simulink model "TRAS_DevDriv"  (R2012b)
settings: Solver=ode4  StartTime=0.0  StopTime=60  FixedStep=0.01  RelTol=1e-3
settings Model: SimulationMode=external  ExtModeTrigDuration=10000  Creator=user  LastModifiedBy=inteco
settings DataIOCC: SignalLoggingSaveFormat=ModelDataLogs
settings DebuggingCC: FcnCallInpInsideContextMsg=UseLocalSettings
settings RTWCC: SystemTargetFile=rtcon_tras_usb2.tlc  TemplateMakefile=rtcon_tras_vc_usb2_x64.tmf  Description=TRAS RTDAC/USB2 (Visual C/C++)  ProcessScript=rtcon_tras_usb2_make_rtw_hook
settings STFCustomTargetCC: CodeReplacementLibrary=ANSI_C  ModelReferenceCompliant=off  GeneratePreprocessorConditionals=Disable all  CombineOutputUpdateFcns=on  MatFileLogging=on  GRTInterface=off  SystemTargetFile=rtcon_tras_usb2.tlc
settings GRTTargetCC: ModelReferenceCompliant=off  ParMdlRefBuildCompliant=off  CompOptLevelCompliant=off  ConcurrentExecutionCompliant=off  ExtMode=on  ExtModeMexFile=rtcon_ext_comm

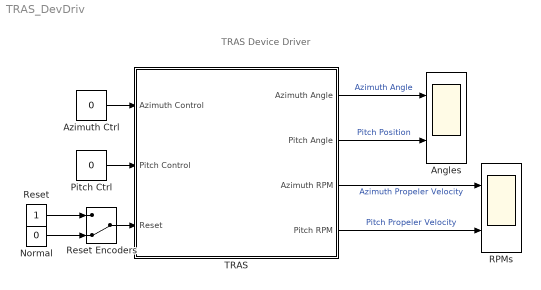
== system TRAS_DevDriv ==
  note: TRAS Device Driver
  Angles : Scope  NumInputPorts=2
      settings: TimeRange=30  YMin=-0.02~-0.1  YMax=0.0025~1  SaveName=SD1  MaxDataPoints=12000
  Azimuth Ctrl : Constant  Value=0
  Normal : Constant  Value=0
  Pitch Ctrl : Constant  Value=0
  RPMs : Scope  NumInputPorts=2
      settings: TimeRange=30  YMin=-20~-400  YMax=0~500  SaveName=SD  MaxDataPoints=12000
  Reset : Constant
  Reset Encoders : ManualSwitch  CurrentSetting=0
  TRAS : Subsystem
      mask Display: image(imread('Tras.JPG'))
  wires:
  TRAS/1(Azimuth Angle) -> Angles/1  "Azimuth Angle"
  TRAS/2(Pitch Angle) -> Angles/2  "Pitch Position"
  Azimuth Ctrl/1 -> TRAS/1(Azimuth Control)
  Pitch Ctrl/1 -> TRAS/2(Pitch Control)
  TRAS/3(Azimuth RPM) -> RPMs/1  "Azimuth Propeler Velocity"
  TRAS/4(Pitch RPM) -> RPMs/2  "Pitch Propeler Velocity"
  Normal/1 -> Reset Encoders/2
  Reset/1 -> Reset Encoders/1
  Reset Encoders/1 -> TRAS/3(Reset)

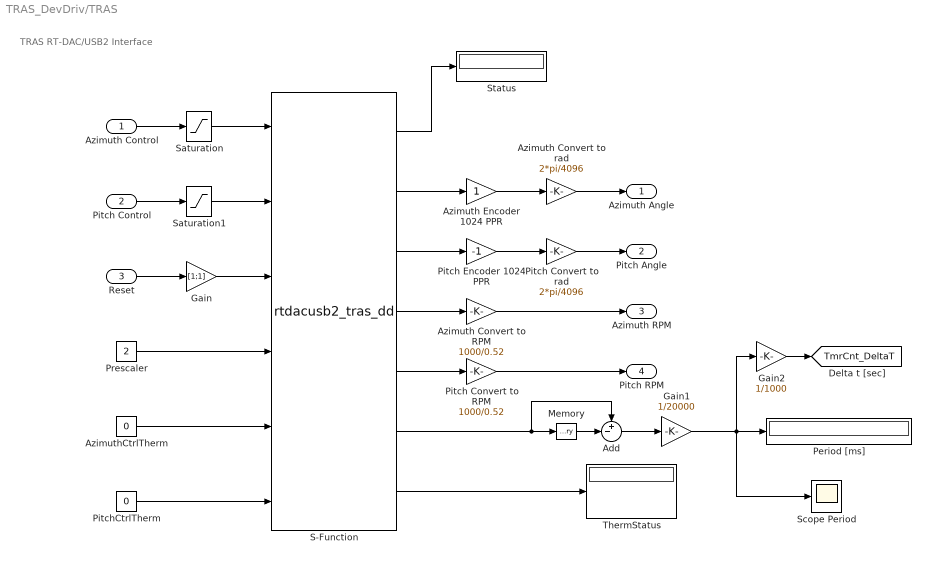
== system TRAS_DevDriv/TRAS ==
  note: TRAS RT-DAC/USB2
      | Interface
  Azimuth Control : Inport
  Pitch Control : Inport  Port=2
  Reset : Inport  Port=3
  Add : Sum  Inputs=+-|
  Azimuth Convert to RPM : Gain  Gain=1000/0.52  SaturateOnIntegerOverflow=on  OutDataTypeStr=Inherit: Same as input  ParamDataTypeStr=Inherit: Same as input
  Azimuth Convert to rad : Gain  Gain=2*pi/4096  SaturateOnIntegerOverflow=on  OutDataTypeStr=Inherit: Same as input  ParamDataTypeStr=Inherit: Same as input
  Azimuth Encoder 1024 PPR : Gain  SaturateOnIntegerOverflow=on  OutDataTypeStr=Inherit: Same as input  ParamDataTypeStr=Inherit: Same as input
  AzimuthCtrlTherm : Constant  Value=0
  Gain : Gain  Gain=[1;1]
  Gain1 : Gain  Gain=1/20000
  Gain2 : Gain  Gain=1/1000
  Memory : Memory
  Period [ms] : Display
  Pitch Convert to RPM : Gain  Gain=1000/0.52  SaturateOnIntegerOverflow=on  OutDataTypeStr=Inherit: Same as input  ParamDataTypeStr=Inherit: Same as input
  Pitch Convert to rad : Gain  Gain=2*pi/4096  SaturateOnIntegerOverflow=on  OutDataTypeStr=Inherit: Same as input  ParamDataTypeStr=Inherit: Same as input
  Pitch Encoder 1024 PPR : Gain  Gain=-1  SaturateOnIntegerOverflow=on  OutDataTypeStr=Inherit: Same as input  ParamDataTypeStr=Inherit: Same as input
  PitchCtrlTherm : Constant  Value=0
  Prescaler : Constant  Value=2
  S-Function : S-Function  FunctionName=rtdacusb2_tras_dd  Parameters=1, 0.01  EnableBusSupport=off
  Saturation : Saturate  UpperLimit=1  LowerLimit=-1
  Saturation1 : Saturate  UpperLimit=1  LowerLimit=-1
  Scope Period : Scope
      settings: TimeRange=30  YMin=0  YMax=6.5e+008
  Status : Display
  ThermStatus : Display
  Azimuth Angle : Outport
  Pitch Angle : Outport  Port=2
  Azimuth RPM : Outport  Port=3
  Pitch RPM : Outport  Port=4
  tag scope: TmrCnt_DeltaT=global
  wires:
  Azimuth Control/1 -> Saturation/1
  Pitch Control/1 -> Saturation1/1
  Reset/1 -> Gain/1
  Prescaler/1 -> S-Function/4
  AzimuthCtrlTherm/1 -> S-Function/5
  PitchCtrlTherm/1 -> S-Function/6
  Saturation/1 -> S-Function/1
  Saturation1/1 -> S-Function/2
  Gain/1 -> S-Function/3
  S-Function/1 -> Status/1
  Azimuth Encoder 1024 PPR/1 -> Azimuth Convert to rad/1
  S-Function/2 -> Azimuth Encoder 1024 PPR/1
  Azimuth Convert to rad/1 -> Azimuth Angle/1
  Pitch Encoder 1024 PPR/1 -> Pitch Convert to rad/1
  S-Function/3 -> Pitch Encoder 1024 PPR/1
  Pitch Convert to rad/1 -> Pitch Angle/1
  S-Function/4 -> Azimuth Convert to RPM/1
  S-Function/5 -> Pitch Convert to RPM/1
  Azimuth Convert to RPM/1 -> Azimuth RPM/1
  Pitch Convert to RPM/1 -> Pitch RPM/1
  S-Function/7 -> ThermStatus/1
  Memory/1 -> Add/2
  Add/1 -> Gain1/1
  S-Function/6 -> Memory/1, Add/1
  Gain1/1 -> Scope Period/1, Period [ms]/1, Gain2/1
  Gain2/1 -> [TmrCnt_DeltaT]
